simulink subsystem "Transmitter"  (R2022b)
settings: Solver=VariableStepAuto  StartTime=0.0  StopTime=10.0  RelTol=1e-3
undefined symbols (not defined in the file or in its folder): debugHeaderGain, G, Rsym
libraries: simulink x44, hdlsllib x29, dspsigops x7, dsphdlfiltering2 x1, whdlmod x1
(part 2 of 2)

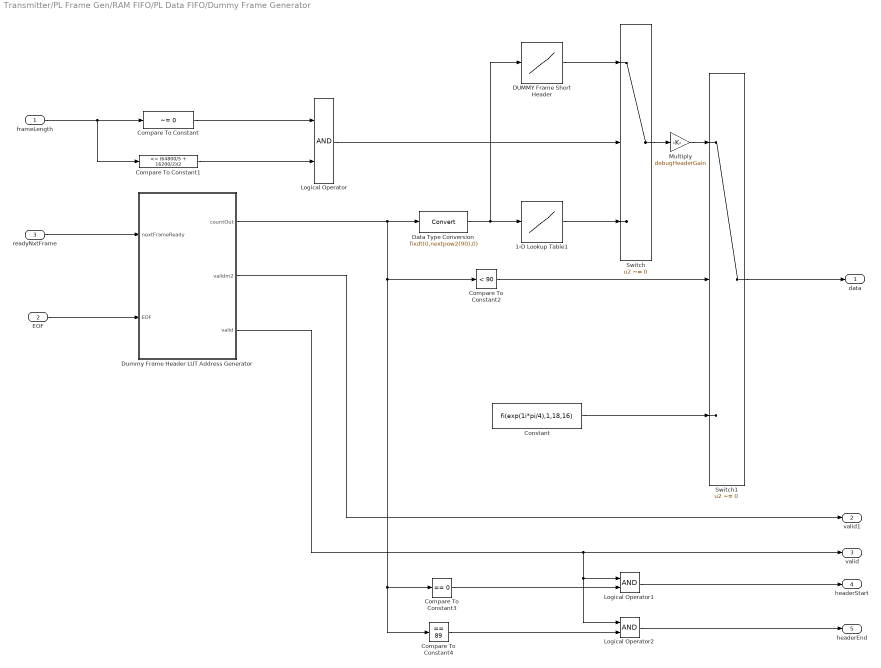
== system Transmitter/PL Frame Gen/RAM FIFO/PL Data FIFO/Dummy Frame Generator ==
  frameLength : Inport
  EOF : Inport  Port=2
  readyNxtFrame : Inport  Port=3
  1-D Lookup Table1 : Lookup_n-D  NumberOfTableDimensions=1  BreakpointsSpecification=Even spacing  BreakpointsForDimension1=[-5:5]  Table="[0.707106781186548 + 0.707106781186548i\t0.707106781186548 - 0.707106781186548i\t-0.707106781186548 - 0.707106781186548i\t-0.707106781186548 + 0.707106781186548i\t0.707106781186548 + 0.707106781186548i\t-0.707106781186548 + 0.707106781186548i\t-0.707106781186548 - 0.707106781186548i\t0.707106781186548 - 0.707106781186548i\t0.707106781186548 + 0.707106781186548i\t0.707106781186548 - 0.707106781186548i\t0.707106781186548 + 0.707106781186548i\t-0.707106781186548 + 0.707106781186548i\t-0.707106781186548 - 0.707106781186548i\t-0.707106781186548 + 0.707106781186548i\t-0.707106781186548 - 0.707106781186548i\t0.707106781186548 - 0.707106781186548i\t-0.707106781186548 - 0.707106781186548i\t-0.707106781186548 + 0.707106781186548i\t-0.707106781186548 - 0.707106781186548i\t-0.707106781186548 + 0.707106781186548i\t0.707106781186548 + 0.707106781186548i\t-0.707106781186548 + 0.707106781186548i\t0.707106781186548 + 0.707106781186548i\t-0.707106781186548 + 0.707106781186548i\t-0.707106781186548 - 0.707106781186548i\t-0.707106781186548 + 0.707106781186548i\t-0.707106781186548 - 0.707106781186548i\t-0.707106781186548 + 0.707106781186548i\t-0.707106781186548 - 0.707106781186548i\t0.707106781186548 - 0.707106781186548i\t-0.707106781186548 - 0.707106781186548i\t0.707106781186548 - 0.707106781186548i\t0.707106781186548 + 0.707106781186548i\t-0.707106781186548 + 0.707106781186548i\t0.707106781186548 + 0.707106781186548i\t-0.707106781186548 + 0.707106781186548i\t0.707106781186548 + 0.707106781186548i\t0.707106781186548 - 0.707106781186548i\t0.707106781186548 + 0.707106781186548i\t-0.707106781186548 + 0.707106781186548i\t0.707106781186548 + 0.707106781186548i\t0.707106781186548 - 0.707106781186548i\t-0.707106781186548 - 0.707106781186548i\t-0.707106781186548 + 0.707106781186548i\t0.707106781186548 + 0.707106781186548i\t-0.707106781186548 + 0.707106781186548i\t0.707106781186548 + 0.707106781186548i\t-0.707106781186548 + 0.707106781186548i\t0.707106781186548 + 0.707106781186548i\t-0.707106781186548 + 0.707106781186548i\t-0.707106781186548 - 0.707106781186548i\t-0.707106781186548 + 0.707106781186548i\t-0.707106781186548 - 0.707106781186548i\t-0.707106781186548 + 0.707106781186548i\t0.707106781186548 + 0.707106781186548i\t0.707106781186548 - 0.707106781186548i\t0.707106781186548 + 0.707106781186548i\t0.707106781186548 - 0.707106781186548i\t0.707106781186548 + 0.707106781186548i\t0.707106781186548 - 0.707106781186548i\t0.707106781186548 + 0.707106781186548i\t0.707106781186548 - 0.707106781186548i\t0.707106781186548 + 0.707106781186548i\t-0.707106781186548 + 0.707106781186548i\t0.707106781186548 + 0.707106781186548i\t0.707106781186548 - 0.707106781186548i\t0.707106781186548 + 0.707106781186548i\t0.707106781186548 - 0.707106781186548i\t-0.707106781186548 - 0.707106781186548i\t0.707106781186548 - 0.707106781186548i\t0.707106781186548 + 0.707106781186548i\t0.707106781186548 - 0.707106781186548i\t-0.707106781186548 - 0.707106781186548i\t0.707106781186548 - 0.707106781186548i\t0.707106781186548 + 0.707106781186548i\t0.707106781186548 - 0.707106781186548i\t0.707106781186548 + 0.707106781186548i\t0.707106781186548 - 0.707106781186548i\t-0.707106781186548 - 0.707106781186548i\t0.707106781186548 - 0.707106781186548i\t0.707106781186548 + 0.707106781186548i\t-0.707106781186548 + 0.707106781186548i\t-0.707106781186548 - 0.707106781186548i\t-0.707106781186548 + 0.707106781186548i\t0.707106781186548 + 0.707106781186548i\t0.707106781186548 - 0.707106781186548i\t-0.707106781186548 - 0.707106781186548i\t0.707106781186548 - 0.707106781186548i\t0.707106781186548 + 0.707106781186548i\t0.707106781186548 - 0.707106781186548i]"  TableDataTypeStr=fixdt(1,18,16)  InterpMethod=Flat  ExtrapMethod=Clip  UseLastTableValue=on  InternalRulePriority=Speed  OutDataTypeStr=fixdt(1,18,16)  RndMeth=Simplest
  Compare To Constant : simulink/Logic and Bit Operations/Compare To Constant  relop=~=  const=0  OutDataTypeStr=boolean
  Compare To Constant1 : simulink/Logic and Bit Operations/Compare To Constant  relop=<=  const=(64800/5 + 16200/2)/2  OutDataTypeStr=boolean
  Compare To Constant2 : simulink/Logic and Bit Operations/Compare To Constant  relop=<  const=90  OutDataTypeStr=boolean
  Compare To Constant3 : simulink/Logic and Bit Operations/Compare To Constant  relop===  const=0  OutDataTypeStr=boolean
  Compare To Constant4 : simulink/Logic and Bit Operations/Compare To Constant  relop===  const=89  OutDataTypeStr=boolean
  Constant : Constant  Value=fi(exp(1i*pi/4),1,18,16)  SampleTime=1/Rsym
  DUMMY Frame Short Header : Lookup_n-D  NumberOfTableDimensions=1  BreakpointsSpecification=Even spacing  BreakpointsForDimension1=[-5:5]  Table="[0.707106781186548 + 0.707106781186548i\t0.707106781186548 - 0.707106781186548i\t-0.707106781186548 - 0.707106781186548i\t-0.707106781186548 + 0.707106781186548i\t0.707106781186548 + 0.707106781186548i\t-0.707106781186548 + 0.707106781186548i\t-0.707106781186548 - 0.707106781186548i\t0.707106781186548 - 0.707106781186548i\t0.707106781186548 + 0.707106781186548i\t0.707106781186548 - 0.707106781186548i\t0.707106781186548 + 0.707106781186548i\t-0.707106781186548 + 0.707106781186548i\t-0.707106781186548 - 0.707106781186548i\t-0.707106781186548 + 0.707106781186548i\t-0.707106781186548 - 0.707106781186548i\t0.707106781186548 - 0.707106781186548i\t-0.707106781186548 - 0.707106781186548i\t-0.707106781186548 + 0.707106781186548i\t-0.707106781186548 - 0.707106781186548i\t-0.707106781186548 + 0.707106781186548i\t0.707106781186548 + 0.707106781186548i\t-0.707106781186548 + 0.707106781186548i\t0.707106781186548 + 0.707106781186548i\t-0.707106781186548 + 0.707106781186548i\t-0.707106781186548 - 0.707106781186548i\t-0.707106781186548 + 0.707106781186548i\t-0.707106781186548 - 0.707106781186548i\t-0.707106781186548 + 0.707106781186548i\t-0.707106781186548 - 0.707106781186548i\t0.707106781186548 - 0.707106781186548i\t-0.707106781186548 - 0.707106781186548i\t0.707106781186548 - 0.707106781186548i\t0.707106781186548 + 0.707106781186548i\t-0.707106781186548 + 0.707106781186548i\t0.707106781186548 + 0.707106781186548i\t-0.707106781186548 + 0.707106781186548i\t0.707106781186548 + 0.707106781186548i\t0.707106781186548 - 0.707106781186548i\t0.707106781186548 + 0.707106781186548i\t-0.707106781186548 + 0.707106781186548i\t0.707106781186548 + 0.707106781186548i\t0.707106781186548 - 0.707106781186548i\t-0.707106781186548 - 0.707106781186548i\t-0.707106781186548 + 0.707106781186548i\t0.707106781186548 + 0.707106781186548i\t-0.707106781186548 + 0.707106781186548i\t0.707106781186548 + 0.707106781186548i\t-0.707106781186548 + 0.707106781186548i\t0.707106781186548 + 0.707106781186548i\t-0.707106781186548 + 0.707106781186548i\t-0.707106781186548 - 0.707106781186548i\t-0.707106781186548 + 0.707106781186548i\t-0.707106781186548 - 0.707106781186548i\t-0.707106781186548 + 0.707106781186548i\t0.707106781186548 + 0.707106781186548i\t0.707106781186548 - 0.707106781186548i\t0.707106781186548 + 0.707106781186548i\t0.707106781186548 - 0.707106781186548i\t-0.707106781186548 - 0.707106781186548i\t-0.707106781186548 + 0.707106781186548i\t-0.707106781186548 - 0.707106781186548i\t-0.707106781186548 + 0.707106781186548i\t-0.707106781186548 - 0.707106781186548i\t0.707106781186548 - 0.707106781186548i\t-0.707106781186548 - 0.707106781186548i\t-0.707106781186548 + 0.707106781186548i\t-0.707106781186548 - 0.707106781186548i\t-0.707106781186548 + 0.707106781186548i\t0.707106781186548 + 0.707106781186548i\t-0.707106781186548 + 0.707106781186548i\t-0.707106781186548 - 0.707106781186548i\t-0.707106781186548 + 0.707106781186548i\t0.707106781186548 + 0.707106781186548i\t-0.707106781186548 + 0.707106781186548i\t-0.707106781186548 - 0.707106781186548i\t-0.707106781186548 + 0.707106781186548i\t-0.707106781186548 - 0.707106781186548i\t-0.707106781186548 + 0.707106781186548i\t0.707106781186548 + 0.707106781186548i\t-0.707106781186548 + 0.707106781186548i\t-0.707106781186548 - 0.707106781186548i\t0.707106781186548 - 0.707106781186548i\t0.707106781186548 + 0.707106781186548i\t0.707106781186548 - 0.707106781186548i\t-0.707106781186548 - 0.707106781186548i\t-0.707106781186548 + 0.707106781186548i\t0.707106781186548 + 0.707106781186548i\t-0.707106781186548 + 0.707106781186548i\t-0.707106781186548 - 0.707106781186548i\t-0.707106781186548 + 0.707106781186548i]"  TableDataTypeStr=fixdt(1,18,16)  InterpMethod=Flat  ExtrapMethod=Clip  UseLastTableValue=on  InternalRulePriority=Speed  OutDataTypeStr=fixdt(1,18,16)  RndMeth=Simplest
  Data Type Conversion : DataTypeConversion  OutDataTypeStr=fixdt(0,nextpow2(90),0)  SaturateOnIntegerOverflow=off  RndMeth=Floor
  Dummy Frame Header LUT Address Generator : MATLAB Function  TreatAsAtomicUnit=on
  Logical Operator : Logic  AllPortsSameDT=off  OutDataTypeStr=boolean
  Logical Operator1 : Logic  AllPortsSameDT=off  OutDataTypeStr=boolean
  Logical Operator2 : Logic  AllPortsSameDT=off  OutDataTypeStr=boolean
  Multiply : Gain  Gain=debugHeaderGain
  Switch : Switch  Criteria=u2 ~= 0  SaturateOnIntegerOverflow=off  InputSameDT=off
  Switch1 : Switch  Criteria=u2 ~= 0  SaturateOnIntegerOverflow=off  InputSameDT=off
  data : Outport
  valid1 : Outport  Port=2
  valid : Outport  Port=3
  headerStart : Outport  Port=4
  headerEnd : Outport  Port=5
  wires:
  Multiply/1 -> Switch1/1
  frameLength/1 -> Compare To Constant1/1, Compare To Constant/1
  Compare To Constant/1 -> Logical Operator/1
  Compare To Constant1/1 -> Logical Operator/2
  Logical Operator/1 -> Switch/2
  DUMMY Frame Short Header/1 -> Switch/1
  1-D Lookup Table1/1 -> Switch/3
  Dummy Frame Header LUT Address Generator/3(valid) -> Logical Operator2/1, Logical Operator1/1, valid/1
  Dummy Frame Header LUT Address Generator/1(countOut) -> Data Type Conversion/1, Compare To Constant4/1, Compare To Constant3/1, Compare To Constant2/1
  Switch/1 -> Multiply/1
  Compare To Constant2/1 -> Switch1/2
  Switch1/1 -> data/1
  Constant/1 -> Switch1/3
  readyNxtFrame/1 -> Dummy Frame Header LUT Address Generator/1(nextFrameReady)
  EOF/1 -> Dummy Frame Header LUT Address Generator/2(EOF)
  Dummy Frame Header LUT Address Generator/2(validm2) -> valid1/1
  Data Type Conversion/1 -> 1-D Lookup Table1/1, DUMMY Frame Short Header/1
  Compare To Constant3/1 -> Logical Operator1/2
  Compare To Constant4/1 -> Logical Operator2/2
  Logical Operator1/1 -> headerStart/1
  Logical Operator2/1 -> headerEnd/1

== system Transmitter/PL Frame Gen/RAM FIFO/PL Data FIFO/Frame Length FIFO ==
  dataIn : Inport
  validIn : Inport  Port=2
  pop : Inport  Port=3
  HDL Counter2 : hdlsllib/Sources/HDL Counter  CountType=Count limited  CountInit=0  CountStep=1  CountMax=2^4 - 1  CountFromType=Initial value  CountFrom=0  CountResetPort=off  CountLoadPort=off  CountEnbPort=on  CountDirPort=off  CountHitOutputPort=off  CountDataType=Unsigned  CountWordLen=4  CountFracLen=0  CountSampTime=1
  HDL Counter3 : hdlsllib/Sources/HDL Counter  CountType=Count limited  CountInit=0  CountStep=1  CountMax=2^4 - 1  CountFromType=Initial value  CountFrom=0  CountResetPort=off  CountLoadPort=off  CountEnbPort=on  CountDirPort=off  CountHitOutputPort=off  CountDataType=Unsigned  CountWordLen=4  CountFracLen=0  CountSampTime=1
  No HDL : Subsystem
  RAM status : MATLAB Function  TreatAsAtomicUnit=on
  Simple Dual Port RAM : hdlsllib/HDL RAMs/Simple Dual Port RAM  ram_size=4
  dataOut : Outport
  wires:
  Simple Dual Port RAM/1 -> dataOut/1
  pop/1 -> RAM status/2(rd), No HDL/5(rd), HDL Counter3/1
  RAM status/2(ncount) -> No HDL/3(ncount)
  HDL Counter2/1 -> Simple Dual Port RAM/2
  dataIn/1 -> Simple Dual Port RAM/1
  HDL Counter3/1 -> Simple Dual Port RAM/4
  RAM status/1(full) -> No HDL/2(full)
  validIn/1 -> RAM status/1(wr), No HDL/1(wr), HDL Counter2/1, Simple Dual Port RAM/3
  RAM status/3(empty) -> No HDL/4(empty)

== system Transmitter/PL Frame Gen/RAM FIFO/PL Data FIFO/No HDL ==
  wr : Inport
  full : Inport  Port=2
  ncount : Inport  Port=3
  empty : Inport  Port=4
  rd : Inport  Port=5
  Assertion : Assertion  AssertionFailFcn=warning('push on to a full RAM');  StopWhenAssertionFail=off
  Assertion1 : Assertion  AssertionFailFcn=warning('pop from an empty RAM');  StopWhenAssertionFail=off
  Display : Display
  Display1 : Display
      settings: Format=decimal (Stored Integer)
  Logical Operator : Logic  Operator=NAND  AllPortsSameDT=off  OutDataTypeStr=boolean
  Logical Operator1 : Logic  Operator=NAND  AllPortsSameDT=off  OutDataTypeStr=boolean
  Subsystem : Subsystem
  wires:
  rd/1 -> Logical Operator1/2
  Logical Operator/1 -> Assertion/1
  empty/1 -> Logical Operator1/1
  ncount/1 -> Subsystem/1(u), Display/1
  full/1 -> Logical Operator/2
  wr/1 -> Logical Operator/1
  Logical Operator1/1 -> Assertion1/1
  Subsystem/1(Out1) -> Display1/1

== system Transmitter/PL Frame Gen/RAM FIFO/PL Header FIFO/monostable 90x ==
  nextFrameReady : Inport
  validOut : Outport
  startOut : Outport  Port=2
  endOut : Outport  Port=3
  endOut1 : Outport  Port=4

== system Transmitter/PL Frame Gen/RAM FIFO/Pilot Generator/Pilot Block Length Valid Generator ==
  trigger : Inport
  Compare To Constant : simulink/Logic and Bit Operations/Compare To Constant  relop===  const=35  OutDataTypeStr=boolean
  Compare To Constant1 : simulink/Logic and Bit Operations/Compare To Constant  relop===  const=34  OutDataTypeStr=boolean
  Compare To Constant2 : simulink/Logic and Bit Operations/Compare To Constant  relop=~=  const=0  OutDataTypeStr=boolean
  HDL Counter : hdlsllib/Sources/HDL Counter  CountType=Count limited  CountInit=0  CountStep=1  CountMax=35  CountFromType=Initial value  CountFrom=0  CountResetPort=off  CountLoadPort=off  CountEnbPort=on  CountDirPort=off  CountHitOutputPort=off  CountDataType=Unsigned  CountWordLen=8  CountFracLen=0  CountSampTime=1
  Logical Operator : Logic  Operator=OR  AllPortsSameDT=off  OutDataTypeStr=boolean
  Scope : Scope  NumInputPorts=3
  endOut : Outport
  endOutm1 : Outport  Port=2
  validOut : Outport  Port=3
  wires:
  Compare To Constant/1 -> Scope/2, endOut/1
  Compare To Constant1/1 -> endOutm1/1
  HDL Counter/1 -> Scope/1, Compare To Constant/1, Compare To Constant2/1, Compare To Constant1/1
  Compare To Constant2/1 -> Logical Operator/2, Scope/3, validOut/1
  trigger/1 -> Logical Operator/1
  Logical Operator/1 -> HDL Counter/1

== system Transmitter/PL Frame Gen/PL Header Generator/PL Header Bits Generator/Header Bits Generator/MODCOD bit number counter ==
  Trigger : Inport
  Constant : Constant  OutDataTypeStr=boolean  SampleTime=-1
  HDL Counter1 : hdlsllib/Sources/HDL Counter  CountType=Count limited  CountInit=0  CountStep=1  CountMax=6  CountFromType=Initial value  CountFrom=0  CountResetPort=on  CountLoadPort=off  CountEnbPort=on  CountDirPort=off  CountHitOutputPort=off  CountDataType=Unsigned  CountWordLen=8  CountFracLen=0  CountSampTime=1
  IsNonZero : simulink/Logic and Bit Operations/Compare To Zero  relop=~=  OutDataTypeStr=boolean
      settings: LibrarySourceBlock=|
      | simulink/Quick Insert/Logic and Bit
      | Operations/IsNonZero
  IsZero : simulink/Logic and Bit Operations/Compare To Zero  relop===  OutDataTypeStr=boolean
      settings: LibrarySourceBlock=|
      | simulink/Quick Insert/Logic and Bit
      | Operations/IsZero
  Logical Operator : Logic  AllPortsSameDT=off  OutDataTypeStr=boolean
  Logical Operator1 : Logic  AllPortsSameDT=off  OutDataTypeStr=boolean
  Logical Operator2 : Logic  Operator=OR  AllPortsSameDT=off  OutDataTypeStr=boolean
  NOT : Logic  Operator=NOT  IconShape=distinctive  AllPortsSameDT=off  OutDataTypeStr=boolean
  NOT1 : Logic  Operator=NOT  IconShape=distinctive  AllPortsSameDT=off  OutDataTypeStr=boolean
  MODCOD bit : Outport
  validOut : Outport  Port=2
  startOfBits : Outport  Port=3
  wires:
  IsZero/1 -> Logical Operator1/2, Logical Operator/1
  HDL Counter1/1 -> MODCOD bit/1, IsNonZero/1, IsZero/1
  Trigger/1 -> NOT/1
  Constant/1 -> HDL Counter1/2
  NOT/1 -> Logical Operator/2
  Logical Operator/1 -> NOT1/1, HDL Counter1/1
  NOT1/1 -> Logical Operator1/1
  Logical Operator1/1 -> Logical Operator2/1, startOfBits/1
  IsNonZero/1 -> Logical Operator2/2
  Logical Operator2/1 -> validOut/1

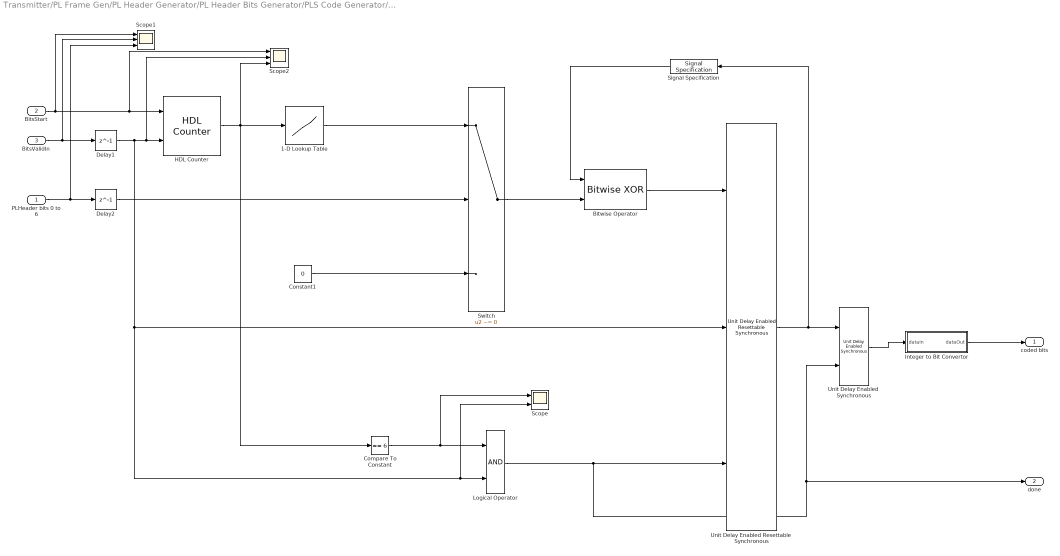
== system Transmitter/PL Frame Gen/PL Header Generator/PL Header Bits Generator/PLS Code Generator/Biorthogonal code ==
  PLHeader bits 0 to 6 : Inport
  BitsStart : Inport  Port=2
  BitsValidIn : Inport  Port=3
  1-D Lookup Table : Lookup_n-D  NumberOfTableDimensions=1  BreakpointsSpecification=Even spacing  BreakpointsForDimension1=[-5:5]  BreakpointsForDimension1FirstPoint=0  Table=[uint32(bit2int(G(1, :).', 32)), uint32(bit2int(G(2, :).', 32)), uint32(bit2int(G(3, :).', 32)), uint32(bit2int(G(4, :).', 32)), uint32(bit2int(G(5, :).', 32)), uint32(bit2int(G(6, :).', 32)), uint32(bit2int(G(7, :).', 32))]  TableDataTypeStr=Inherit: Inherit from 'Table data'  InterpMethod=Flat  DiagnosticForOutOfRangeInput=Warning  InternalRulePriority=Speed  OutDataTypeStr=Inherit: Inherit from 'Table data'  RndMeth=Simplest
  Bitwise Operator : simulink/Logic and Bit Operations/Bitwise Operator  logicop=XOR  UseBitMask=off  NumInputPorts=2  BitMask=bin2dec('11011001')  BitMaskRealWorld=Stored Integer
  Compare To Constant : simulink/Logic and Bit Operations/Compare To Constant  relop===  const=6  OutDataTypeStr=boolean
  Constant1 : Constant  Value=0  OutDataTypeStr=uint32  SampleTime=2/(Rsym)
  Delay1 : Delay  DelayLength=1
  Delay2 : Delay  DelayLength=1
  HDL Counter : hdlsllib/Sources/HDL Counter  CountType=Count limited  CountInit=0  CountStep=1  CountMax=6  CountFromType=Initial value  CountFrom=0  CountResetPort=on  CountLoadPort=off  CountEnbPort=on  CountDirPort=off  CountHitOutputPort=off  CountDataType=Unsigned  CountWordLen=nextpow2(5)  CountFracLen=0  CountSampTime=1
  Integer to Bit Convertor : Subsystem
  Logical Operator : Logic  AllPortsSameDT=off  OutDataTypeStr=boolean
  Scope : Scope  NumInputPorts=2
  Scope1 : Scope  NumInputPorts=3
  Scope2 : Scope  NumInputPorts=3
  Signal Specification : SignalSpecification  OutDataTypeStr=uint32
  Switch : Switch  Criteria=u2 ~= 0  SaturateOnIntegerOverflow=off  InputSameDT=off
  Unit Delay Enabled Synchronous : hdlsllib/Discrete/Unit Delay Enabled Synchronous  InitialCondition=0.0  SampleTime=-1
  Unit Delay Enabled Resettable Synchronous : hdlsllib/Discrete/Unit Delay Enabled Resettable Synchronous  InitialCondition=0.0  SampleTime=-1
  coded bits : Outport
  done : Outport  Port=2
  wires:
  BitsStart/1 -> Scope1/1, Scope2/1, HDL Counter/1
  HDL Counter/1 -> Compare To Constant/1, Scope2/3, 1-D Lookup Table/1
  BitsValidIn/1 -> Delay1/1, Scope1/2
  1-D Lookup Table/1 -> Switch/1
  PLHeader bits 0 to 6/1 -> Delay2/1, Scope1/3
  Constant1/1 -> Switch/3
  Logical Operator/1 -> done/1, Unit Delay Enabled Synchronous/2, Unit Delay Enabled Resettable Synchronous/3
  Compare To Constant/1 -> Scope/1, Logical Operator/1
  Unit Delay Enabled Resettable Synchronous/1 -> Signal Specification/1, Unit Delay Enabled Synchronous/1
  Unit Delay Enabled Synchronous/1 -> Integer to Bit Convertor/1(dataIn)
  Integer to Bit Convertor/1(dataOut) -> coded bits/1
  Switch/1 -> Bitwise Operator/2
  Bitwise Operator/1 -> Unit Delay Enabled Resettable Synchronous/1
  Signal Specification/1 -> Bitwise Operator/1
  Delay1/1 -> Scope/2, Logical Operator/2, Unit Delay Enabled Resettable Synchronous/2, Scope2/2, HDL Counter/2
  Delay2/1 -> Switch/2

== system Transmitter/PL Frame Gen/PL Header Generator/PL Header Bits Generator/PLS Code Generator/PLSC Scrambler ==
  bits in : Inport
  resetIn : Inport  Port=2
  validIn1 : Inport  Port=3
  1-D Lookup Table : Lookup_n-D  NumberOfTableDimensions=1  LookupTableObject=''  BreakpointsSpecification=Even spacing  BreakpointsForDimension1=[-5:5]  BreakpointsForDimension1FirstPoint=0  BreakpointsForDimension2FirstPoint=10  BreakpointsForDimension2Spacing=12  IndexSearchMethod=Evenly spaced points  Table=[1 0 1 1 1 1 0 0 0 0 0 1 0 0 0 1 1 0 0 0 0 0 0 0 1 0 1 0 0 1 0 1 0 1 0 1 0 0 0 1 0 1 1 1 0 1 1 1 0 1 0 1 1 1 0 0 1 0 0 1 1 1 0 1 1 0 0 0 0 1 0 1 1 0 0 0 1 1 1 1 1 1 0 1 1 0 1 0 1 1 0 0 1 1 0 1 1 0 1 1 1 0 0 0 0 1 1 1 0 0 0 1 1 0 1 0 1 0 0 1 1 1 1 1 0 0 0 1 0 0 0 0 1 1 0 0 1 0 1 0 0 0 0 0 0 1 1 1 1 0 1 1 1 1]  InterpMethod=Flat  DiagnosticForOutOfRangeInput=Error  InternalRulePriority=Speed  RndMeth=Simplest
  Compare To Constant : simulink/Logic and Bit Operations/Compare To Constant  relop===  const=63  OutDataTypeStr=boolean
  Data Type Conversion : DataTypeConversion  OutDataTypeStr=boolean  SaturateOnIntegerOverflow=off  RndMeth=Floor
  Delay : Delay  DelayLength=1
  Delay1 : Delay  DelayLength=1
  Delay2 : Delay
  Delay3 : Delay  DelayLength=1
  Logical Operator : Logic  Operator=XOR  AllPortsSameDT=off  OutDataTypeStr=boolean
  Logical Operator1 : Logic  AllPortsSameDT=off  OutDataTypeStr=boolean
  PLSC Valid Counter : hdlsllib/Sources/HDL Counter  CountType=Free running  CountInit=0  CountStep=1  CountMax=154-1  CountFromType=Initial value  CountFrom=0  CountResetPort=on  CountLoadPort=off  CountEnbPort=on  CountDirPort=off  CountHitOutputPort=off  CountDataType=Unsigned  CountWordLen=8  CountFracLen=0  CountSampTime=1
  Scope : Scope  NumInputPorts=4
  Scope1 : Scope  NumInputPorts=3
  Scope2 : Scope  NumInputPorts=3
  DataOut : Outport
  EndOfPLSC : Outport  Port=2
  ValidOut : Outport  Port=3
  wires:
  PLSC Valid Counter/1 -> Scope/3, Compare To Constant/1, 1-D Lookup Table/1
  Data Type Conversion/1 -> Scope2/1, Logical Operator/2
  Logical Operator1/1 -> Scope1/2, EndOfPLSC/1
  Logical Operator/1 -> Scope2/3, Scope1/1, DataOut/1
  validIn1/1 -> Delay/1
  resetIn/1 -> Scope/4, PLSC Valid Counter/1
  Delay/1 -> Delay1/1, Delay3/1, PLSC Valid Counter/2
  Compare To Constant/1 -> Scope/1, Logical Operator1/1
  Delay1/1 -> Scope/2, Logical Operator1/2
  bits in/1 -> Delay2/1
  1-D Lookup Table/1 -> Data Type Conversion/1
  Delay2/1 -> Scope2/2, Logical Operator/1
  Delay3/1 -> Scope1/3, ValidOut/1

== system Transmitter/PL Frame Gen/PL Header Generator/PL Header Bits Generator/PLS Code Generator/Serializer ==
  coded bits : Inport
  trigger : Inport  Port=2
  Compare To Constant : simulink/Logic and Bit Operations/Compare To Constant  relop===  const=1  OutDataTypeStr=boolean
  Compare To Constant1 : simulink/Logic and Bit Operations/Compare To Constant  relop=~=  const=1  OutDataTypeStr=boolean
  Constant : Constant  OutDataTypeStr=boolean  SampleTime=-1
  Demux : Demux  Commented=on  Outputs=32
  HDL Counter : hdlsllib/Sources/HDL Counter  CountType=Count limited  CountInit=1  CountStep=1  CountMax=32  CountFromType=Initial value  CountFrom=1  CountResetPort=on  CountLoadPort=off  CountEnbPort=on  CountDirPort=off  CountHitOutputPort=off  CountDataType=Unsigned  CountWordLen=8  CountFracLen=0  CountSampTime=-1
  Logical Operator : Logic  AllPortsSameDT=off  OutDataTypeStr=boolean
  Logical Operator1 : Logic  AllPortsSameDT=off  OutDataTypeStr=boolean
  Logical Operator2 : Logic  Operator=OR  AllPortsSameDT=off  OutDataTypeStr=boolean
  Multiport Switch : MultiPortSwitch  Commented=on  Inputs=32  SaturateOnIntegerOverflow=off  InputSameDT=off
  NOT : Logic  Operator=NOT  IconShape=distinctive  AllPortsSameDT=off  OutDataTypeStr=boolean
  NOT1 : Logic  Operator=NOT  IconShape=distinctive  AllPortsSameDT=off  OutDataTypeStr=boolean
  Scope : Scope  NumInputPorts=4
  CodedBits1_7 : Outport
  startOut : Outport  Port=2
  validOut : Outport  Port=3
  wires:
  HDL Counter/1 -> Compare To Constant1/1, Scope/3, Compare To Constant/1
  Constant/1 -> HDL Counter/2
  trigger/1 -> NOT1/1
  NOT/1 -> Logical Operator1/1
  NOT1/1 -> Logical Operator/1
  Logical Operator1/1 -> Logical Operator2/1, Scope/1, startOut/1
  Compare To Constant/1 -> Logical Operator/2, Logical Operator1/2
  Logical Operator/1 -> NOT/1, HDL Counter/1
  Compare To Constant1/1 -> Logical Operator2/2
  Logical Operator2/1 -> Scope/2, validOut/1
  Demux/27 -> Multiport Switch/28
  Demux/29 -> Multiport Switch/30
  Demux/23 -> Multiport Switch/24
  Demux/24 -> Multiport Switch/25
  Demux/32 -> Multiport Switch/33
  Demux/30 -> Multiport Switch/31
  Demux/25 -> Multiport Switch/26
  Multiport Switch/1 -> ?
  Demux/15 -> Multiport Switch/16
  Demux/22 -> Multiport Switch/23
  Demux/18 -> Multiport Switch/19
  Demux/13 -> Multiport Switch/14
  Demux/26 -> Multiport Switch/27
  Demux/16 -> Multiport Switch/17
  ? -> Multiport Switch/1
  Demux/11 -> Multiport Switch/12
  Demux/21 -> Multiport Switch/22
  Demux/31 -> Multiport Switch/32
  Demux/12 -> Multiport Switch/13
  Demux/9 -> Multiport Switch/10
  Demux/14 -> Multiport Switch/15
  Demux/2 -> Multiport Switch/3
  Demux/5 -> Multiport Switch/6
  Demux/6 -> Multiport Switch/7
  Demux/8 -> Multiport Switch/9
  Demux/20 -> Multiport Switch/21
  Demux/1 -> Multiport Switch/2
  Demux/19 -> Multiport Switch/20
  Demux/10 -> Multiport Switch/11
  Demux/3 -> Multiport Switch/4
  Demux/28 -> Multiport Switch/29
  Demux/17 -> Multiport Switch/18
  Demux/7 -> Multiport Switch/8
  Demux/4 -> Multiport Switch/5
  coded bits/1 -> CodedBits1_7/1

== system Transmitter/PL Frame Gen/PL Header Generator/PL Header Bits Generator/PLS Code Generator/Serializer1 ==
  coded bits : Inport
  trigger : Inport  Port=2
  Compare To Constant : simulink/Logic and Bit Operations/Compare To Constant  relop=~=  const=0  OutDataTypeStr=boolean
  Compare To Constant1 : simulink/Logic and Bit Operations/Compare To Constant  relop===  const=31  OutDataTypeStr=boolean
  Demux : Demux  Outputs=32
  HDL Counter : hdlsllib/Sources/HDL Counter  CountType=Count limited  CountInit=0  CountStep=1  CountMax=31  CountFromType=Initial value  CountFrom=0  CountResetPort=on  CountLoadPort=off  CountEnbPort=on  CountDirPort=off  CountHitOutputPort=off  CountDataType=Unsigned  CountWordLen=8  CountFracLen=0  CountSampTime=1
  Logical Operator : Logic  Operator=OR  AllPortsSameDT=off  OutDataTypeStr=boolean
  Multiport Switch : MultiPortSwitch  DataPortOrder=Zero-based contiguous  Inputs=32  zeroidx=on  SaturateOnIntegerOverflow=off  InputSameDT=off
  Scope : Scope  NumInputPorts=3
  CodedBits1_7 : Outport
  startOut : Outport  Port=2
  validOut : Outport  Port=3
  wires:
  Demux/27 -> Multiport Switch/28
  Demux/29 -> Multiport Switch/30
  Demux/23 -> Multiport Switch/24
  Demux/24 -> Multiport Switch/25
  Demux/32 -> Multiport Switch/33
  Demux/30 -> Multiport Switch/31
  Demux/25 -> Multiport Switch/26
  Multiport Switch/1 -> Scope/1, CodedBits1_7/1
  Demux/15 -> Multiport Switch/16
  Demux/22 -> Multiport Switch/23
  Demux/18 -> Multiport Switch/19
  Demux/13 -> Multiport Switch/14
  Demux/26 -> Multiport Switch/27
  Demux/16 -> Multiport Switch/17
  HDL Counter/1 -> Compare To Constant1/1, Compare To Constant/1, Multiport Switch/1
  Demux/11 -> Multiport Switch/12
  Demux/21 -> Multiport Switch/22
  Demux/31 -> Multiport Switch/32
  Demux/12 -> Multiport Switch/13
  Demux/9 -> Multiport Switch/10
  Demux/14 -> Multiport Switch/15
  Demux/2 -> Multiport Switch/3
  Demux/5 -> Multiport Switch/6
  Demux/6 -> Multiport Switch/7
  Demux/8 -> Multiport Switch/9
  Demux/20 -> Multiport Switch/21
  Demux/1 -> Multiport Switch/2
  Demux/19 -> Multiport Switch/20
  Demux/10 -> Multiport Switch/11
  Demux/3 -> Multiport Switch/4
  Demux/28 -> Multiport Switch/29
  Demux/17 -> Multiport Switch/18
  Demux/7 -> Multiport Switch/8
  Demux/4 -> Multiport Switch/5
  coded bits/1 -> Demux/1
  trigger/1 -> Scope/2, startOut/1, Logical Operator/2
  Compare To Constant/1 -> Logical Operator/1
  Compare To Constant1/1 -> HDL Counter/1
  Logical Operator/1 -> Scope/3, validOut/1, HDL Counter/2

== system Transmitter/PL Frame Gen/PL Header Generator/PL Header Bits Generator/SOF Generator/SOF Length Counter ==
  Trigger : Inport
  Constant : Constant  OutDataTypeStr=boolean  SampleTime=-1
  HDL Counter1 : hdlsllib/Sources/HDL Counter  CountType=Count limited  CountInit=0  CountStep=1  CountMax=25  CountFromType=Initial value  CountFrom=0  CountResetPort=on  CountLoadPort=off  CountEnbPort=on  CountDirPort=off  CountHitOutputPort=on  CountDataType=Unsigned  CountWordLen=8  CountFracLen=0  CountSampTime=1
  IsNonZero : simulink/Logic and Bit Operations/Compare To Zero  relop=~=  OutDataTypeStr=boolean
      settings: LibrarySourceBlock=|
      | simulink/Quick Insert/Logic and Bit
      | Operations/IsNonZero
  IsZero : simulink/Logic and Bit Operations/Compare To Zero  relop===  OutDataTypeStr=boolean
      settings: LibrarySourceBlock=|
      | simulink/Quick Insert/Logic and Bit
      | Operations/IsZero
  Logical Operator : Logic  AllPortsSameDT=off  OutDataTypeStr=boolean
  Logical Operator1 : Logic  AllPortsSameDT=off  OutDataTypeStr=boolean
  Logical Operator2 : Logic  Operator=OR  AllPortsSameDT=off  OutDataTypeStr=boolean
  NOT : Logic  Operator=NOT  IconShape=distinctive  AllPortsSameDT=off  OutDataTypeStr=boolean
  NOT1 : Logic  Operator=NOT  IconShape=distinctive  AllPortsSameDT=off  OutDataTypeStr=boolean
  Scope : Scope  Commented=on  NumInputPorts=3
  LUT address : Outport
  validOut : Outport  Port=2
  StartOfOSOF : Outport  Port=3
  wires:
  IsZero/1 -> Logical Operator1/2, Logical Operator/1
  Trigger/1 -> NOT/1
  Constant/1 -> HDL Counter1/2
  NOT/1 -> Logical Operator/2
  Logical Operator/1 -> NOT1/1, HDL Counter1/1
  IsNonZero/1 -> Logical Operator2/2
  NOT1/1 -> Logical Operator1/1
  Logical Operator1/1 -> Scope/3, Logical Operator2/1, StartOfOSOF/1
  HDL Counter1/1 -> Scope/1, LUT address/1, IsNonZero/1, IsZero/1
  Logical Operator2/1 -> Scope/2, validOut/1

== system Transmitter/PL Frame Gen/RAM FIFO/PL Data FIFO/Frame Length FIFO/No HDL ==
  wr : Inport
  full : Inport  Port=2
  ncount : Inport  Port=3
  empty : Inport  Port=4
  rd : Inport  Port=5
  Assertion : Assertion  AssertionFailFcn=warning('pop from an empty RAM');  StopWhenAssertionFail=off
  Assertion1 : Assertion  AssertionFailFcn=warning('push on to a full RAM');  StopWhenAssertionFail=off
  Display : Display
  Display1 : Display
  Logical Operator : Logic  Operator=NAND  AllPortsSameDT=off  OutDataTypeStr=boolean
  Logical Operator1 : Logic  Operator=NAND  AllPortsSameDT=off  OutDataTypeStr=boolean
  Subsystem : Subsystem
  wires:
  wr/1 -> Logical Operator/1
  full/1 -> Logical Operator/2
  ncount/1 -> Subsystem/1(u), Display/1
  empty/1 -> Logical Operator1/1
  rd/1 -> Logical Operator1/2
  Logical Operator/1 -> Assertion1/1
  Logical Operator1/1 -> Assertion/1
  Subsystem/1(Out1) -> Display1/1

== system Transmitter/PL Frame Gen/RAM FIFO/PL Data FIFO/No HDL/Subsystem ==
  u : Inport
  Relational Operator : RelationalOperator  Operator=>  OutDataTypeStr=boolean  RndMeth=Simplest  InputSameDT=off
  Unit Delay Enabled Synchronous : hdlsllib/Discrete/Unit Delay Enabled Synchronous  InitialCondition=0.0  SampleTime=-1
  Out1 : Outport
  wires:
  Unit Delay Enabled Synchronous/1 -> Out1/1, Relational Operator/2
  u/1 -> Unit Delay Enabled Synchronous/1, Relational Operator/1
  Relational Operator/1 -> Unit Delay Enabled Synchronous/2

== system Transmitter/PL Frame Gen/PL Header Generator/PL Header Bits Generator/PLS Code Generator/Biorthogonal code/Integer to Bit Convertor ==
  dataIn : Inport
  For Each Subsystem : Subsystem  TreatAsAtomicUnit=on
  For Each Subsystem1 : Subsystem  TreatAsAtomicUnit=on
  For Each Subsystem2 : Subsystem  TreatAsAtomicUnit=on
  For Each Subsystem3 : Subsystem  TreatAsAtomicUnit=on
  Subsystem : Subsystem
  dataOut : Outport
  wires:
  Subsystem/1(Out1) -> For Each Subsystem/1(In1)
  For Each Subsystem2/1(Out1) -> For Each Subsystem3/1(In1)
  For Each Subsystem1/1(Out1) -> For Each Subsystem2/1(In1)
  For Each Subsystem/1(Out1) -> For Each Subsystem1/1(In1)
  dataIn/1 -> Subsystem/2(u1), Subsystem/1(u)
  For Each Subsystem3/1(Out1) -> dataOut/1

== system Transmitter/PL Frame Gen/RAM FIFO/PL Data FIFO/Frame Length FIFO/No HDL/Subsystem ==
  u : Inport
  Relational Operator : RelationalOperator  Operator=>  OutDataTypeStr=boolean  RndMeth=Simplest  InputSameDT=off
  Unit Delay Enabled Synchronous : hdlsllib/Discrete/Unit Delay Enabled Synchronous  InitialCondition=0.0  SampleTime=-1
  Out1 : Outport
  wires:
  Unit Delay Enabled Synchronous/1 -> Out1/1, Relational Operator/2
  u/1 -> Unit Delay Enabled Synchronous/1, Relational Operator/1
  Relational Operator/1 -> Unit Delay Enabled Synchronous/2

== system Transmitter/PL Frame Gen/PL Header Generator/PL Header Bits Generator/PLS Code Generator/Biorthogonal code/Integer to Bit Convertor/For Each Subsystem ==
  In1 : Inport  Partition=on  PartitionDimension=1  PartitionWidth=1  PartitionOffset=0
  Extract Bits2 : simulink/Logic and Bit Operations/Extract Bits  bitsToExtract=Upper half  numBits=8  bitIdxRange=[32 63]  outScalingMode=Treat bit field as an integer
  Extract Bits3 : simulink/Logic and Bit Operations/Extract Bits  bitsToExtract=Lower half  numBits=8  bitIdxRange=[32 63]  outScalingMode=Treat bit field as an integer
  For Each : ForEach  DisableCoverage=on
  Mux1 : Mux  Inputs=2
  Out1 : Outport  ConcatenationDimension=1
  wires:
  Extract Bits3/1 -> Mux1/2
  In1/1 -> Extract Bits2/1, Extract Bits3/1
  Extract Bits2/1 -> Mux1/1
  Mux1/1 -> Out1/1

== system Transmitter/PL Frame Gen/PL Header Generator/PL Header Bits Generator/PLS Code Generator/Biorthogonal code/Integer to Bit Convertor/For Each Subsystem1 ==
  In1 : Inport  Partition=on  PartitionDimension=1  PartitionWidth=1  PartitionOffset=0
  Extract Bits2 : simulink/Logic and Bit Operations/Extract Bits  bitsToExtract=Upper half  numBits=8  bitIdxRange=[32 63]  outScalingMode=Treat bit field as an integer
  Extract Bits3 : simulink/Logic and Bit Operations/Extract Bits  bitsToExtract=Lower half  numBits=8  bitIdxRange=[32 63]  outScalingMode=Treat bit field as an integer
  For Each : ForEach  DisableCoverage=on
  Mux1 : Mux  Inputs=2
  Out1 : Outport  ConcatenationDimension=1
  wires:
  Mux1/1 -> Out1/1
  Extract Bits2/1 -> Mux1/1
  In1/1 -> Extract Bits3/1, Extract Bits2/1
  Extract Bits3/1 -> Mux1/2

== system Transmitter/PL Frame Gen/PL Header Generator/PL Header Bits Generator/PLS Code Generator/Biorthogonal code/Integer to Bit Convertor/For Each Subsystem2 ==
  In1 : Inport  Partition=on  PartitionDimension=1  PartitionWidth=1  PartitionOffset=0
  Extract Bits2 : simulink/Logic and Bit Operations/Extract Bits  bitsToExtract=Upper half  numBits=8  bitIdxRange=[32 63]  outScalingMode=Treat bit field as an integer
  Extract Bits3 : simulink/Logic and Bit Operations/Extract Bits  bitsToExtract=Lower half  numBits=8  bitIdxRange=[32 63]  outScalingMode=Treat bit field as an integer
  For Each : ForEach  DisableCoverage=on
  Mux1 : Mux  Inputs=2
  Out1 : Outport  ConcatenationDimension=1
  wires:
  Extract Bits3/1 -> Mux1/2
  In1/1 -> Extract Bits2/1, Extract Bits3/1
  Extract Bits2/1 -> Mux1/1
  Mux1/1 -> Out1/1

== system Transmitter/PL Frame Gen/PL Header Generator/PL Header Bits Generator/PLS Code Generator/Biorthogonal code/Integer to Bit Convertor/For Each Subsystem3 ==
  In1 : Inport  Partition=on  PartitionDimension=1  PartitionWidth=1  PartitionOffset=0
  Extract Bits2 : simulink/Logic and Bit Operations/Extract Bits  bitsToExtract=Upper half  numBits=8  bitIdxRange=[32 63]  outScalingMode=Treat bit field as an integer
  Extract Bits3 : simulink/Logic and Bit Operations/Extract Bits  bitsToExtract=Lower half  numBits=8  bitIdxRange=[32 63]  outScalingMode=Treat bit field as an integer
  For Each : ForEach  DisableCoverage=on
  Mux1 : Mux  Inputs=2
  Out1 : Outport  ConcatenationDimension=1
  wires:
  Mux1/1 -> Out1/1
  Extract Bits2/1 -> Mux1/1
  In1/1 -> Extract Bits3/1, Extract Bits2/1
  Extract Bits3/1 -> Mux1/2

== system Transmitter/PL Frame Gen/PL Header Generator/PL Header Bits Generator/PLS Code Generator/Biorthogonal code/Integer to Bit Convertor/Subsystem ==
  u : Inport
  u1 : Inport  Port=2
  Extract Bits2 : simulink/Logic and Bit Operations/Extract Bits  bitsToExtract=Upper half  numBits=8  bitIdxRange=[32 63]  outScalingMode=Treat bit field as an integer
  Extract Bits3 : simulink/Logic and Bit Operations/Extract Bits  bitsToExtract=Lower half  numBits=8  bitIdxRange=[32 63]  outScalingMode=Treat bit field as an integer
  Mux1 : Mux  Inputs=2
  Out1 : Outport
  wires:
  Mux1/1 -> Out1/1
  u1/1 -> Extract Bits3/1
  u/1 -> Extract Bits2/1
  Extract Bits3/1 -> Mux1/2
  Extract Bits2/1 -> Mux1/1

== matlab function Transmitter/PL Frame Gen/RAM FIFO/PL Data FIFO/RAM status ==
  data: full output; ncount output; wr input; empty output; rd input
function [full,ncount,empty] = fcn(wr,rd)
%#codegen
     
    WL = 16;
    persistent count;
    if isempty(count)
        count = fi(0,0,WL+1,0,hdlfimath);
    end

    empty = (count == 0);
    full = (count > 2^WL-1);
    ncount = count;

    if wr
        count(:) = count + 1;
    end
    if rd
        count(:) = count - 1;
    end

end

== matlab function Transmitter/PL Frame Gen/RAM FIFO/PL Data FIFO/Out Frame Count ==
  data: startOutFrame output; endOutFrame output; endOutFramem2 output; endOut16Slots output; validOut output; endOfPLHeader input; endOfPilotBlk input; frameLength input
function [startOutFrame,endOutFrame,endOutFramem2,endOut16Slots,validOut] = counter(endOfPLHeader,endOfPilotBlk,frameLength)
%#codegen

   LENGTH = 90*16;
   persistent slotCount countActive slotEnd frameCount;
   if isempty(slotCount)
       slotCount = fi(0,0,nextpow2(LENGTH -1),0);
       countActive = false;
       slotEnd = false;
       frameCount = cast(0,'like',frameLength);
   end
   
   endOut16Slots = slotEnd;
   validOut = countActive;
   endOutFrame = countActive && (frameCount == frameLength-1);
   endOutFramem2 = countActive && (frameCount == frameLength-1-2);
   startOutFrame = countActive && (frameCount == 0);

   if countActive && (frameCount == frameLength-1)
       slotCount(:) = 0;
       countActive = false;
       slotEnd = false;
       frameCount(:) = 0;
   else
       if countActive
           frameCount(:) = frameCount + 1;
           if slotCount == LENGTH-1
               slotCount(:) = 0;
               countActive = false;
           else
               slotCount(:) = slotCount + 1;
           end
           if slotCount == LENGTH-1
               slotEnd = true;
           else
               slotEnd = false;
           end
       else
           slotEnd = false;
       end

       if (endOfPLHeader && (frameCount == 0)) || (endOfPilotBlk && (frameCount ~= 0))
           countActive = true;
       end
   end

end

== matlab function Transmitter/PL Frame Gen/Multiplexer/Priority Encoder ==
  data: x1 input; y output; x2 input; x3 input; x4 input
function y = fcn(x1,x2,x3,x4)
%#codegen

  if x4
    y = fi(3,0,2,0);
  elseif x3
      y = fi(2,0,2,0);
  elseif x2
      y = fi(1,0,2,0);
  else
      y = fi(0,0,2,0);
  end

end

== matlab function Transmitter/PL Frame Gen/RAM FIFO/PL Data FIFO/In Frame Count ==
  data: countOut output; enb input; endOut output; countToValue input
function [countOut,endOut] = counter(enb,countToValue)
%#codegen

   persistent count;
   if isempty(count)
       count = cast(0,'like',countToValue);
   end
   
   countOut = count;
   if countToValue == 0
       endOut = false;
   else
       endOut = (count == countToValue-1) && enb;
   end

   if enb
       if (count ~= 0) && (count == countToValue-1)
           count(:) = 0;
       else
           count(:) = count + 1;
       end
   end

end

== matlab function Transmitter/PL Frame Gen/RAM FIFO/Pilot Generator/Pilot Block Length Valid Generator1 ==
  data: endOut output; endOutm1 output; trigger input; validOut output
function [endOut,endOutm1,validOut] = monostable(trigger)
%#codegen

   LENGTH = 36;
   persistent count countActive countEnd countEndm1;
   if isempty(count)
       count = fi(0,0,nextpow2(LENGTH -1),0);
       countActive = false;
       countEnd = false;
       countEndm1 = false;
   end
   
   endOut = countEnd;
   validOut = countActive;
   endOutm1 = countEndm1;

   if countActive
       if count == LENGTH-1
           count(:) = 0;
           countActive = false;
       else
           count(:) = count + 1;
       end
       if count == LENGTH-2
           countEndm1 = true;
       else
           countEndm1 = false;
       end
       if count == LENGTH-1
           countEnd = true;
       else
           countEnd = false;
       end
   else
       countEnd = false;
       countEndm1 = false;
   end


   if trigger
       countActive = true;
   end

end

== matlab function Transmitter/PL Frame Gen/RAM FIFO/PL Header FIFO/90x ==
  data: validOut output; startOut output; endOut output; trigger input; endOutm1 output
function [validOut,startOut,endOut,endOutm1] = monostable(trigger)
%#codegen
   
   LENGTH = 90;
   persistent count countActive;
   if isempty(count)
       count = fi(0,0,nextpow2(LENGTH-1),0);
       countActive = false;
   end
   
   validOut = countActive;
   endOut = (count == LENGTH-1) && countActive;
   endOutm1 = (count == LENGTH-2) && countActive;
   startOut = (count == 0) && countActive;

   if countActive
       if count == LENGTH-1
           count(:) = 0;
           countActive = false;
       else
           count(:) = count + 1;
       end
   end

   if trigger
       countActive = true;
   end

end

== matlab function Transmitter/PL Frame Gen/RAM FIFO/PL Data FIFO/Dummy Frame Generator/Dummy Frame Header LUT Address Generator ==
  data: countOut output; validm2 output; nextFrameReady input; valid output; EOF input
function [countOut,validm2,valid] = fcn(nextFrameReady,EOF)
%#codegen
  
  dummyFrameLength = 90 + 36*90;
  persistent count countActive;
  if isempty(count)
      count = fi(0,0,nextpow2(dummyFrameLength - 1),0,hdlfimath);
      countActive = false;
  end

  if ~countActive && EOF && ~nextFrameReady
      countActive = true;
  end

  valid = countActive;
  validm2 = countActive && (count<=dummyFrameLength-3);
  countOut = count;
  
  if countActive
      if count == dummyFrameLength-1
          count(:) = 0;
          countActive = false;
      else
          count(:) = count + 1;
      end
  end

end

== matlab function Transmitter/PL Frame Gen/RAM FIFO/PL Data FIFO/Frame Length FIFO/RAM status ==
  data: full output; ncount output; wr input; empty output; rd input
function [full,ncount,empty] = fcn(wr,rd)
%#codegen
     
    WL = 4;
    persistent count;
    if isempty(count)
        count = fi(0,0,WL+1,0,hdlfimath);
    end

    empty = (count == 0);
    full = (count > 2^WL-1);
    ncount = count;

    if wr
        count(:) = count + 1;
    end
    if rd
        count(:) = count - 1;
    end

end
